simulink model "flybackkk"  (R2017b)
settings: Solver=FixedStepAuto  StartTime=0.0  StopTime=0.1  FixedStep=1e-7  MaxStep=1e-4  MinStep=1e-11  RelTol=1e-4
libraries: powerlib x29, powerlib_meascontrol x4
settings Model: Creator=tunay  LastModifiedBy=user
settings CodeAppCC: StateflowObjectComments=on
settings SimscapeCC: SimscapeNormalizeSystem=off

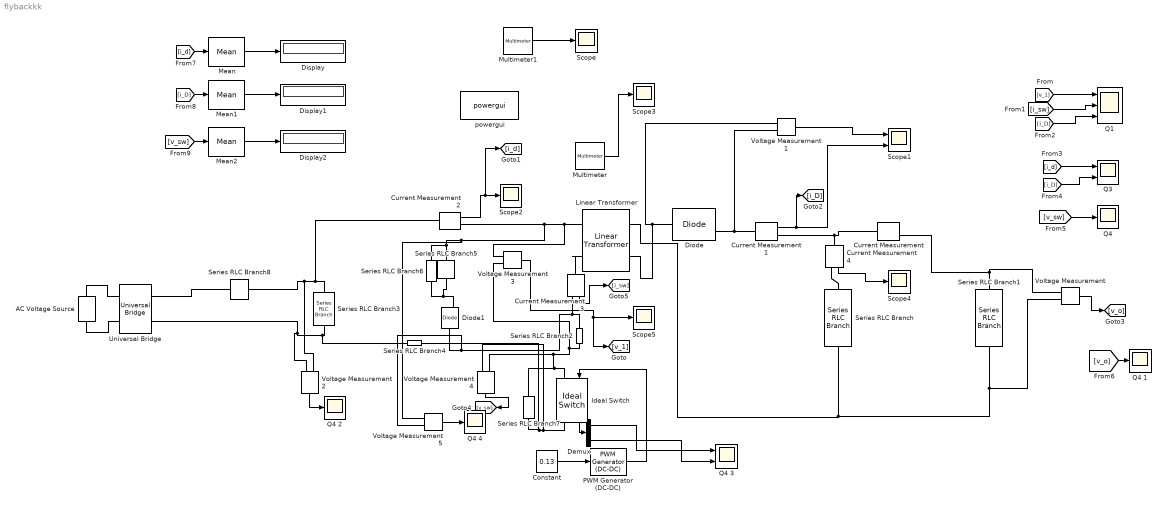
== system flybackkk ==
  AC Voltage Source : powerlib/Electrical Sources/AC Voltage Source  Amplitude=265*sqrt(2)  Phase=0  Frequency=50  SampleTime=1e-7  Measurements=None  BusType=swing  Pref=10e3  Qref=0  Qmin=-inf  Qmax=+inf
  Constant : Constant  Value=0.13
  Current Measurement{,1..4} (5 alike) : powerlib/Measurements/Current Measurement  PhasorSimulation=off  OutputType=Complex  PSBequivalent=0
  Demux : Demux  Outputs=2
  Diode : powerlib/Power Electronics/Diode  Ron=0.001  Lon=0  Vf=0.8  IC=0  UseSnubber=0  Rs=500  Cs=250e-9  Measurements=on
  Diode1 : powerlib/Power Electronics/Diode  Ron=0.001  Lon=0  Vf=0.8  IC=0  UseSnubber=0  Rs=inf  Cs=0  Measurements=on
  Display : Display
  Display1 : Display
  Display2 : Display
  Ideal Switch : powerlib/Power Electronics/Ideal Switch  Ron=0.6e-3  Lon=0  IC=0  Rs=1e3  Cs=1e-12  Measurements=on
  Linear Transformer : powerlib/Elements/Linear Transformer  UNITS=SI  NominalPower="[ 55  40e3 ]"  winding1=[120 0 0]  winding2=[120*0.25 0 0]  ThreeWindings=off  winding3=[3.15e+05 1.323e+06 105.28]  RmLm=[1e6 618e-6]  Measurements=Winding currents  DataType=on
  Mean : powerlib_meascontrol/Measurements/Mean  Freq=100e3  Vinit=0  Ts=0
  Mean1 : powerlib_meascontrol/Measurements/Mean  Freq=100e3  Vinit=0  Ts=0
  Mean2 : powerlib_meascontrol/Measurements/Mean  Freq=100e3  Vinit=0  Ts=0
  Multimeter : powerlib/Measurements/Multimeter  PhasorSimulation=off  OutputType=Complex  sel=3  L=4  Gain=1  yselected={'Iw1: Linear Transformer'};  PSBOutputType=1  PSBequivalent=0  AxesSetting=[0,0.1,-100,100]  Display=0  SavedBlockNames=-11
  Multimeter1 : powerlib/Measurements/Multimeter  PhasorSimulation=off  OutputType=Complex  sel=[1 2]  L=4  Gain=[1 1]  yselected={'Ub: Series RLC Branch5','Ib: Series RLC Branch5'};  PSBOutputType=1  PSBequivalent=0  AxesSetting=[0,0.1,-100,100]  Display=0  SavedBlockNames=-11
  PWM Generator (DC-DC) : powerlib_meascontrol/Pulse & Signal Generators/PWM Generator (DC-DC)  Fsw=40e3  Ts=1e-7
  "Q1 " : Scope  NumInputPorts=3
  "Q3 " : Scope  NumInputPorts=2
  Q4 {,1..2,4} (4 alike) : Scope
  Q4 3 : Scope  NumInputPorts=2
  Scope{,2..5} (5 alike) : Scope
  Scope1 : Scope  NumInputPorts=2
  Series RLC Branch : powerlib/Elements/Series RLC Branch  LConnTagsString=__new0  RConnTagsString=__new0  BranchType=C  Resistance=1  Inductance=1e-3  SetiL0=off  InitialCurrent=0  Capacitance=200e-6  Setx0=off  InitialVoltage=15  Measurements=None
  Series RLC Branch1 : powerlib/Elements/Series RLC Branch  LConnTagsString=__new0  RConnTagsString=__new0  BranchType=R  Resistance=12  Inductance=1e-3  SetiL0=off  InitialCurrent=0  Capacitance=1e-6  Setx0=off  InitialVoltage=0  Measurements=None
  Series RLC Branch2 : powerlib/Elements/Series RLC Branch  LConnTagsString=__new0  RConnTagsString=__new0  BranchType=L  Resistance=12  Inductance=1e-7  SetiL0=off  InitialCurrent=0  Capacitance=1e-6  Setx0=off  InitialVoltage=0  Measurements=None
  Series RLC Branch3 : powerlib/Elements/Series RLC Branch  LConnTagsString=__new0  RConnTagsString=__new0  BranchType=RC  Resistance=10e-3  Inductance=1e-3  SetiL0=off  InitialCurrent=0  Capacitance=220e-6  Setx0=off  InitialVoltage=15  Measurements=None
  Series RLC Branch4 : powerlib/Elements/Series RLC Branch  LConnTagsString=__new0  RConnTagsString=__new0  BranchType=L  Resistance=12  Inductance=1e-7  SetiL0=off  InitialCurrent=0  Capacitance=1e-6  Setx0=off  InitialVoltage=0  Measurements=None
  Series RLC Branch5 : powerlib/Elements/Series RLC Branch  LConnTagsString=__new0  RConnTagsString=__new0  BranchType=R  Resistance=150  Inductance=1e-3  SetiL0=off  InitialCurrent=0  Capacitance=5e-3  Setx0=off  InitialVoltage=15  Measurements=Branch voltage and current
  Series RLC Branch6 : powerlib/Elements/Series RLC Branch  LConnTagsString=__new0  RConnTagsString=__new0  BranchType=C  Resistance=10e-3  Inductance=1e-3  SetiL0=off  InitialCurrent=0  Capacitance=4.471e-9  Setx0=off  InitialVoltage=15  Measurements=None
  Series RLC Branch7 : powerlib/Elements/Series RLC Branch  LConnTagsString=__new0  RConnTagsString=__new0  BranchType=C  Resistance=10e-3  Inductance=1e-3  SetiL0=off  InitialCurrent=0  Capacitance=9e-12  Setx0=off  InitialVoltage=15  Measurements=None
  Series RLC Branch8 : powerlib/Elements/Series RLC Branch  LConnTagsString=__new0  RConnTagsString=__new0  BranchType=L  Resistance=12  Inductance=44e-6  SetiL0=off  InitialCurrent=0  Capacitance=1e-6  Setx0=off  InitialVoltage=0  Measurements=None
  Universal Bridge : powerlib/Power Electronics/Universal Bridge  Arms=2  SnubberResistance=1e5  SnubberCapacitance=inf  Device=Diodes  Ron=1e-3  Lon=0  ForwardVoltages="[  0  0  ]"  ForwardVoltage=0.7  GTOparameters=[ 10e-6 , 20e-6 ]  IGBTparameters=[ 1e-6 , 2e-6 ]  Measurements=None  Measurements_2=None  converterType=Rectifier
  Voltage Measurement{,1..5} (6 alike) : powerlib/Measurements/Voltage Measurement  PhasorSimulation=off  OutputType=Complex  PSBequivalent=0
  powergui : powerlib/powergui  Priority=1  SimulationMode=Discrete  SampleTime=1e-7  frequency=60  Iterations=50  frequencyindice=0  Pbase=100e6  ErrMax=1e-4  UnitsV=kV  UnitsW=MW  buscounter=0  FunctionMessages=off  echomessages=off  EnableUseOfTLC=off  CurrentSourceSwitches=off  DisableSnubberDevices=off  DisableRonSwitches=off  DisableVfSwitches=off  DisplayEquations=off  SolverType=Tustin/Backward Euler (TBE)  Interpol=off  ExternalGateDelay=off  methode=off  Ts=100  x0status=blocks  SPID=off  SwTol=0  HookPort=off  RestoreLinks=warning  ResistiveCurrentMeasurement=off  Frange=[0:2:500]  Ylog=off  Xlog=on  ShowGrid=off  save=off  variable=ZData  structure=0  ZoomFFT=off  StartTime=0.0  cycles=1  DisplayStyle=1  fundamental=60  FreqAxis=off  MaxFrequency=1000  frequencyindicesteady=1  RmsSteady=1  display=off
  wires:
  PWM Generator (DC-DC)/1 -> Ideal Switch/1
  Constant/1 -> PWM Generator (DC-DC)/1
  Voltage Measurement/1 -> [v_o]
  Voltage Measurement1/1 -> Scope1/1
  Current Measurement1/1 -> [i_D], Scope1/2
  Current Measurement2/1 -> [i_d], Scope2/1
  Multimeter/1 -> Scope3/1
  Voltage Measurement3/1 -> [v_1], Scope5/1
  Voltage Measurement4/1 -> [v_sw]
  [v_1] -> "Q1 "/1
  [i_D] -> "Q1 "/3
  [i_sw] -> "Q1 "/2
  [i_d] -> "Q3 "/1
  [i_D] -> "Q3 "/2
  [v_sw] -> "Q4 "/1
  [v_o] -> Q4 1/1
  Current Measurement3/1 -> [i_sw]
  [i_d] -> Mean/1
  [i_D] -> Mean1/1
  Mean/1 -> Display/1
  Mean1/1 -> Display1/1
  Mean2/1 -> Display2/1
  [v_sw] -> Mean2/1
  Voltage Measurement2/1 -> Q4 2/1
  Ideal Switch/1 -> Demux/1
  Demux/1 -> Q4 3/1
  Demux/2 -> Q4 3/2
  Voltage Measurement5/1 -> Q4 4/1
  Current Measurement4/1 -> Scope4/1
  Multimeter1/1 -> Scope/1
  connections:
  Voltage Measurement1/LConn1 -- Diode/LConn1 -- Linear Transformer/RConn2
  Series RLC Branch/RConn1 -- Linear Transformer/RConn1 -- Voltage Measurement/LConn2 -- Series RLC Branch1/RConn1
  Voltage Measurement/LConn1 -- Current Measurement/RConn1 -- Series RLC Branch1/LConn1
  Current Measurement1/RConn1 -- Current Measurement4/LConn1 -- Current Measurement/LConn1
  Current Measurement1/LConn1 -- Voltage Measurement1/LConn2 -- Diode/RConn1
  Current Measurement2/RConn1 -- Voltage Measurement5/LConn1 -- Series RLC Branch6/RConn1 -- Series RLC Branch5/LConn1 -- Linear Transformer/LConn1 -- Voltage Measurement3/LConn1
  Linear Transformer/LConn2 -- Current Measurement3/LConn1
  Voltage Measurement3/LConn2 -- Series RLC Branch2/RConn1 -- Series RLC Branch7/RConn1 -- Ideal Switch/LConn1 -- Voltage Measurement4/LConn1
  Series RLC Branch2/LConn1 -- Voltage Measurement5/LConn2 -- Diode1/LConn1 -- Current Measurement3/RConn1
  AC Voltage Source/RConn1 -- Universal Bridge/LConn1
  AC Voltage Source/LConn1 -- Universal Bridge/LConn2
  Universal Bridge/RConn1 -- Series RLC Branch8/RConn1
  Series RLC Branch3/RConn1 -- Series RLC Branch4/RConn1 -- Voltage Measurement2/LConn2 -- Universal Bridge/RConn2
  Voltage Measurement4/LConn2 -- Series RLC Branch7/LConn1 -- Series RLC Branch4/LConn1 -- Ideal Switch/RConn1
  Diode1/RConn1 -- Series RLC Branch6/LConn1 -- Series RLC Branch5/RConn1
  Current Measurement4/RConn1 -- Series RLC Branch/LConn1
  Series RLC Branch8/LConn1 -- Voltage Measurement2/LConn1 -- Current Measurement2/LConn1 -- Series RLC Branch3/LConn1
